simulink model "Position_Control_Test"  (R2017b)
settings: Solver=VariableStepAuto  StartTime=0.0  StopTime=30  RelTol=1e-3
undefined symbols (not defined in the file): psi, x, y, z
libraries: NLGCToolbox x4
settings Model: Creator=hoang  LastModifiedBy=hoang

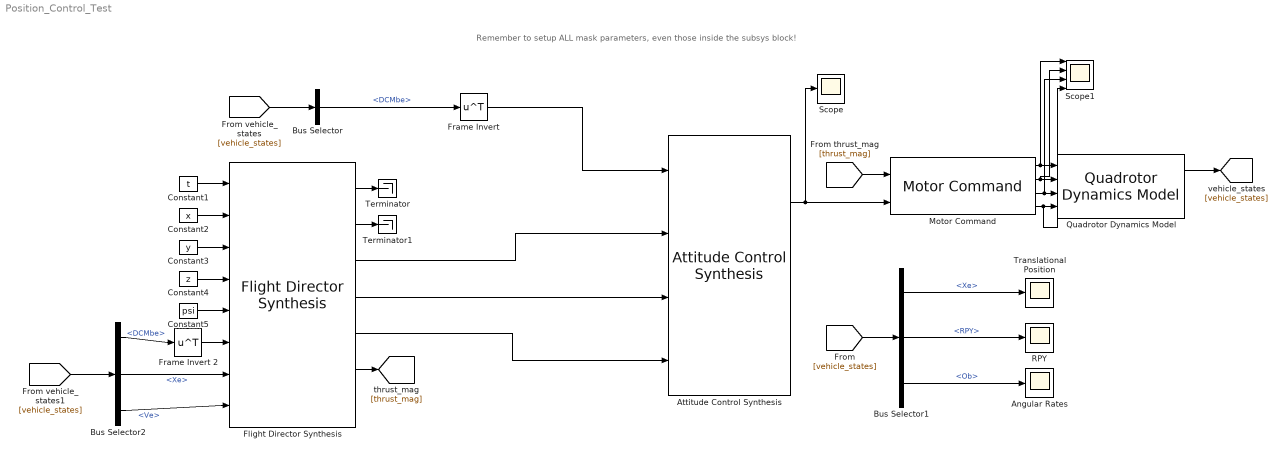
== system Position_Control_Test ==
  note: Remember to setup ALL mask parameters, even those inside the subsys block!
  Angular Rates : Scope
  Attitude Control Synthesis : NLGCToolbox/Attitude Control Synthesis  quadrotor=quad  Ts1=1/120
      settings: SourceProductName=Thinh - NLGC for Quadrotor
  Bus Selector : BusSelector  OutputSignals=DCMbe
  Bus Selector1 : BusSelector  OutputSignals=Xe,RPY,Ob
  Bus Selector2 : BusSelector  OutputSignals=DCMbe,Xe,Ve
  Constant1 : Constant  Value=t
  Constant2 : Constant  Value=x
  Constant3 : Constant  Value=y
  Constant4 : Constant  Value=z
  Constant5 : Constant  Value=psi
  Flight Director Synthesis : NLGCToolbox/Flight Director Synthesis  Ts=1/120  kx=64  kv=42  xinit=[0;0;-4]  quadrotor=quad
      settings: SourceProductName=Thinh - NLGC for Quadrotor
  Frame Invert : Math  Operator=transpose  SaturateOnIntegerOverflow=on
  Frame Invert 2 : Math  Operator=transpose  SaturateOnIntegerOverflow=on
  Motor Command : NLGCToolbox/Motor Command  quadrotor=quad
      settings: SourceProductName=Thinh - NLGC for Quadrotor
  Quadrotor Dynamics Model : NLGCToolbox/Quadrotor Dynamics Model  xinit=[0;0;-4]  quadrotor=quad
      settings: SourceProductName=Thinh - NLGC for Quadrotor
  RPY : Scope
  Scope : Scope
  Scope1 : Scope  NumInputPorts=4
  Terminator : Terminator
  Terminator1 : Terminator
  Translational Position : Scope
  wires:
  Motor Command/1 -> Scope1/1, Quadrotor Dynamics Model/1
  Motor Command/2 -> Scope1/2, Quadrotor Dynamics Model/2
  Motor Command/3 -> Scope1/3, Quadrotor Dynamics Model/3
  Motor Command/4 -> Scope1/4, Quadrotor Dynamics Model/4
  Quadrotor Dynamics Model/1 -> [vehicle_states]
  [vehicle_states] -> Bus Selector/1
  Bus Selector/1 -> Frame Invert/1  "<DCMbe>"
  Frame Invert/1 -> Attitude Control Synthesis/1
  Flight Director Synthesis/3 -> Attitude Control Synthesis/2
  Flight Director Synthesis/4 -> Attitude Control Synthesis/3
  [vehicle_states] -> Bus Selector1/1
  Bus Selector1/2 -> RPY/1  "<RPY>"
  Bus Selector1/3 -> Angular Rates/1  "<Ob>"
  Bus Selector1/1 -> Translational Position/1  "<Xe>"
  Attitude Control Synthesis/1 -> Scope/1, Motor Command/2
  Constant1/1 -> Flight Director Synthesis/1
  Constant2/1 -> Flight Director Synthesis/2
  Constant3/1 -> Flight Director Synthesis/3
  Constant4/1 -> Flight Director Synthesis/4
  Constant5/1 -> Flight Director Synthesis/5
  [vehicle_states] -> Bus Selector2/1
  Frame Invert 2/1 -> Flight Director Synthesis/6
  Bus Selector2/1 -> Frame Invert 2/1  "<DCMbe>"
  Bus Selector2/2 -> Flight Director Synthesis/7  "<Xe>"
  Bus Selector2/3 -> Flight Director Synthesis/8  "<Ve>"
  Flight Director Synthesis/5 -> Attitude Control Synthesis/4
  Flight Director Synthesis/1 -> Terminator/1
  Flight Director Synthesis/2 -> Terminator1/1
  Flight Director Synthesis/6 -> [thrust_mag]
  [thrust_mag] -> Motor Command/1
